simulink model "Reactortestmdl"  (R2020a)
settings: Solver=VariableStepAuto  StartTime=0.0  StopTime=10  RelTol=1e-3
settings Model: Creator=marce  LastModifiedBy=marce
settings DataIOCC: ReturnWorkspaceOutputs=off

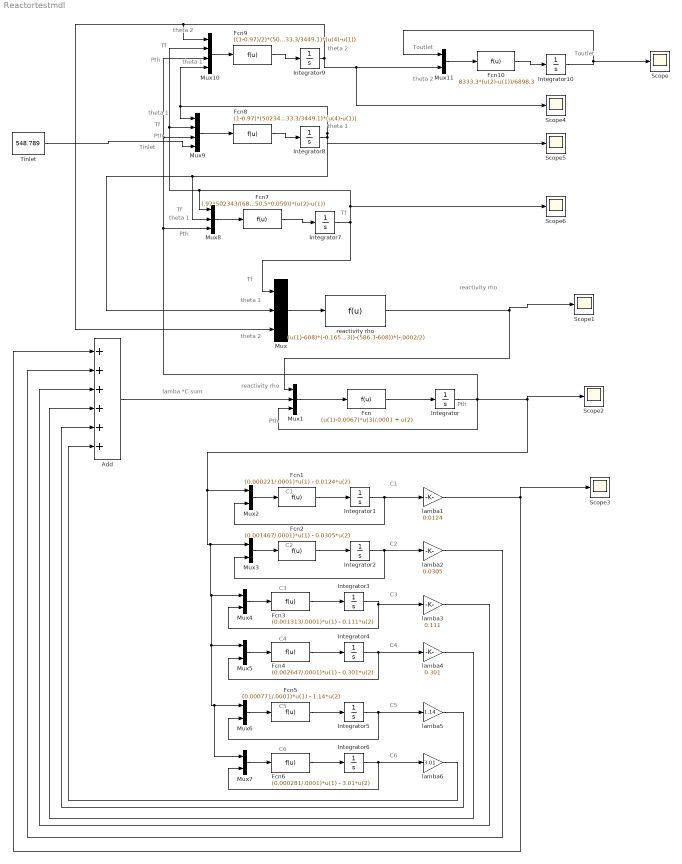
== system Reactortestmdl ==
  note: Tinlet
  note: Pth
  note: theta 1
  note: Tf
  note: C1
  note: lamba *C sum
  note: Pth
  note: reactivity rho
  note: theta 2
  note: theta 1
  note: Tf
  note: reactivity rho
  note: Pth
  note: C2
  note: C3
  note: C4
  note: C5
  note: C6
  note: C1
  note: C2
  note: C3
  note: C4
  note: C5
  note: C6
  note: Tf
  note: theta 1
  note: theta 1
  note: Tf
  note: Pth
  note: theta 2
  note: theta 2
  note: Tf
  note: Pth
  note: theta 1
  note: theta 2
  note: Toutlet
  note: Toutlet
  Add : Sum  Inputs=++++++
  Fcn : Fcn  Expr=(u(1)-0.0067)*u(3)/.0001 + u(2)
  Fcn1 : Fcn  Expr=(0.000221/.0001)*u(1) - 0.0124*u(2)
  Fcn10 : Fcn  Expr=8333.3*(u(2)-u(1))/6898.3
  Fcn2 : Fcn  Expr=(0.001467/.0001)*u(1) - 0.0305*u(2)
  Fcn3 : Fcn  Expr=(0.001313/.0001)*u(1) - 0.111*u(2)
  Fcn4 : Fcn  Expr=(0.002647/.0001)*u(1) - 0.301*u(2)
  Fcn5 : Fcn  Expr=(0.000771/.0001)*u(1) - 1.14*u(2)
  Fcn6 : Fcn  Expr=(0.000281/.0001)*u(1) - 3.01*u(2)
  Fcn7 : Fcn  Expr=(.97*502343/(6898.3*0.059))*u(3) + (0.0909*14120.6/(53850.5*0.059))*(u(2)-u(1))
  Fcn8 : Fcn  Expr=(1-0.97)*(502343/(3449.1*1.376))*u(3)+(0.0909*7060.3/(3449.1*1.376))*(u(2)-u(1))+(8333.3/3449.1)*(u(4)-u(1))
  Fcn9 : Fcn  Expr=((1-0.97)/2)*(502343/(3449.1*1.376))*u(3)+(0.0909*7060.3/(3449.1*1.376))*(u(2)-u(4))+(8333.3/3449.1)*(u(4)-u(1))
  Integrator : Integrator  InitialCondition=.001
  Integrator{1..10} (10 alike) : Integrator
  Mux : Mux  Inputs=3
  Mux1 : Mux  Inputs=3
  Mux10 : Mux
  Mux{2..7,11} (7 alike) : Mux  Inputs=2
  Mux8 : Mux  Inputs=3
  Mux9 : Mux
  Scope{,1..6} (7 alike) : Scope
  Tinlet : Constant  Value=548.789
  lamba1 : Gain  Gain=0.0124
  lamba2 : Gain  Gain=0.0305
  lamba3 : Gain  Gain=0.111
  lamba4 : Gain  Gain=0.301
  lamba5 : Gain  Gain=1.14
  lamba6 : Gain  Gain=3.01
  reactivity rho : Fcn  Expr=(u(1)-608)*(-0.165e-5)+((u(2)-u(3))-(586.3-608))*(-.0002/2)
  wires:
  Fcn/1 -> Integrator/1
  Mux1/1 -> Fcn/1
  Integrator/1 -> Mux1/3, Mux7/1, Mux6/1, Mux5/1, Mux4/1, Mux3/1, Mux2/1, Scope2/1, Mux9/3, Mux10/3, Mux8/3
  Mux2/1 -> Fcn1/1
  Fcn1/1 -> Integrator1/1
  Integrator1/1 -> lamba1/1, Mux2/2
  Fcn2/1 -> Integrator2/1
  Integrator2/1 -> Mux3/2, lamba2/1
  Mux3/1 -> Fcn2/1
  Fcn3/1 -> Integrator3/1
  Integrator3/1 -> lamba3/1, Mux4/2
  Mux4/1 -> Fcn3/1
  Fcn4/1 -> Integrator4/1
  Integrator4/1 -> lamba4/1, Mux5/2
  Mux5/1 -> Fcn4/1
  Fcn5/1 -> Integrator5/1
  Integrator5/1 -> lamba5/1, Mux6/2
  Mux6/1 -> Fcn5/1
  Fcn6/1 -> Integrator6/1
  Integrator6/1 -> lamba6/1, Mux7/2
  Mux7/1 -> Fcn6/1
  lamba1/1 -> Add/1, Scope3/1
  lamba6/1 -> Add/6
  lamba5/1 -> Add/5
  lamba4/1 -> Add/4
  lamba3/1 -> Add/3
  lamba2/1 -> Add/2
  Mux8/1 -> Fcn7/1
  Fcn7/1 -> Integrator7/1
  Integrator7/1 -> Mux10/2, Mux9/2, Mux8/1, Scope6/1, Mux/1
  Fcn8/1 -> Integrator8/1
  Integrator8/1 -> Mux10/4, Mux9/1, Scope5/1, Mux/2, Mux8/2
  Mux9/1 -> Fcn8/1
  Fcn9/1 -> Integrator9/1
  Mux10/1 -> Fcn9/1
  Integrator9/1 -> Mux10/1, Mux/3, Scope4/1, Mux11/2
  Fcn10/1 -> Integrator10/1
  Integrator10/1 -> Scope/1, Mux11/1
  Mux11/1 -> Fcn10/1
  Tinlet/1 -> Mux9/4
  Mux/1 -> reactivity rho/1
  Add/1 -> Mux1/2
  reactivity rho/1 -> Scope1/1, Mux1/1
